simulink model "freq_lookup_table"  (R2015b)
settings: Solver=VariableStepAuto  StartTime=0.0  StopTime=25  RelTol=1e-3
undefined symbols (not defined in the file or in its folder): freq, time, Ts
libraries: powerlib x1
settings Model: Creator=Eren  LastModifiedBy=Eren

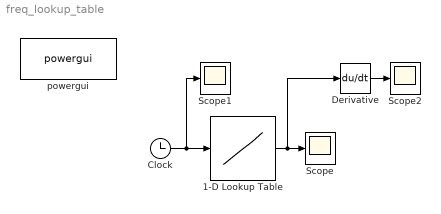
== system freq_lookup_table ==
  1-D Lookup Table : Lookup_n-D  NumberOfTableDimensions=1  BreakpointsForDimension1=time  Table=freq  InternalRulePriority=Speed  RndMeth=Simplest  InputSameDT=on
  Clock : Clock
      settings: Decimation=100000000
  Derivative : Derivative
  Scope : Scope
  Scope1 : Scope
  Scope2 : Scope
  powergui : powerlib/powergui  Priority=2  SimulationMode=Discrete  SolverType=Tustin  SampleTime=Ts  frequency=60  SPID=off  DisableSnubberDevices=off  DisableRonSwitches=off  DisableVfSwitches=off  SwTol=0  DisplayEquations=off  Interpol=off  ExternalGateDelay=off  methode=off  Ts=0  FunctionMessages=off  echomessages=off  HookPort=off  EnableUseOfTLC=off  x0status=blocks  frequencyindice=50  Pbase=100e6  ErrMax=1e-4  Iterations=50  UnitsV=kV  UnitsW=MW  buscounter=0  RestoreLinks=warning  ResistiveCurrentMeasurement=off  Frange=[0:2:500]  Ylog=off  Xlog=on  ShowGrid=off  save=off  variable=ZData  structure=0  ZoomFFT=on  StartTime=0.0  cycles=1  DisplayStyle=1  fundamental=60  FreqAxis=off  MaxFrequency=1000  frequencyindicesteady=1  RmsSteady=1  display=off
  wires:
  1-D Lookup Table/1 -> Derivative/1, Scope/1
  Clock/1 -> Scope1/1, 1-D Lookup Table/1
  Derivative/1 -> Scope2/1
